simulink subsystem "TController"  (R2021a)
settings: Solver=VariableStepAuto  StartTime=0.0  StopTime=10.0  RelTol=1e-3
(part 1 of 2)
settings Model: Creator=phill  LastModifiedBy=phill

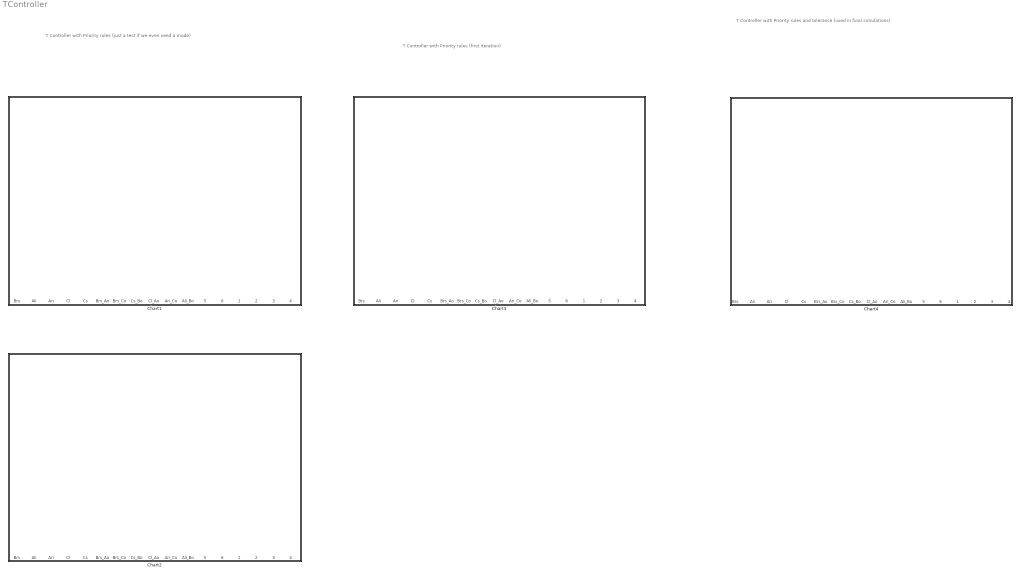
== system TController ==
  note: T Controller with Priority rules (first iteration)
  note: T Controller with Priority rules (just a test if we even need a mode)
  note: T Controller with Priority rules and tolerance
      | (used in final simulations)
  Chart1 : Stateflow chart  TreatAsAtomicUnit=on
      settings: PortSchema="{\"entries\":[{\"content\":{\"sides\":[{\"content\":{\"connectorIds\":[]},\"type\":\"ConnectorPlacement.EquallySpacedRectSide\",\"uuid\":\"dee1a780-e9dd-4205-adb9-3e9cb1ec0cd6\"},{\"content\":{\"connectorIds\":[],\"side\":\"RIGHT\"},\"type\":\"ConnectorPlacement.EquallySpacedRectSide\",\"uuid\":\"bc6af08d-2df8-4a74-93d0-032b7c1c381c\"},{\"content\":{\"connectorIds\":[],\"side\":\"TOP\"},\"type\":\"ConnectorPlacement.EquallySpacedRectSide\",\"uuid\":\"98fea325-c9fc-472d-8e1a-d846d6e99e12\"},{\"content\":{\"connectorIds\":[\"In5\",\"In1\",\"In2\",\"In3\",\"In4\",\"In11\",\"In10\",\"In9\",\"In8\",\"In7\",\"In6\",\"Out5\",\"Out6\",\"Out1\",\"Out2\",\"Out3\",\"Out4\"],\"side\":\"BOTTOM\"},\"type\":\"ConnectorPlacement.EquallySpacedRectSide\",\"uuid\":\"a092283f-ef46-48e2-a5f8-8210ac00b2f9\"}]},\"type\":\"ConnectorPlacement.EquallySpacedConnector\",\"uuid\":\"33a851aa-4180-41c0-b4bb-9b9c3be41936\"}],\"packageUris\":[\"http://schema.mathworks.com/mf0/Connector/R2020b\"],\"version\":\"1.0\"}"
  Chart2 : Stateflow chart  TreatAsAtomicUnit=on
      settings: PortSchema="{\"entries\":[{\"content\":{\"sides\":[{\"content\":{\"connectorIds\":[]},\"type\":\"ConnectorPlacement.EquallySpacedRectSide\",\"uuid\":\"dee1a780-e9dd-4205-adb9-3e9cb1ec0cd6\"},{\"content\":{\"connectorIds\":[],\"side\":\"RIGHT\"},\"type\":\"ConnectorPlacement.EquallySpacedRectSide\",\"uuid\":\"bc6af08d-2df8-4a74-93d0-032b7c1c381c\"},{\"content\":{\"connectorIds\":[],\"side\":\"TOP\"},\"type\":\"ConnectorPlacement.EquallySpacedRectSide\",\"uuid\":\"98fea325-c9fc-472d-8e1a-d846d6e99e12\"},{\"content\":{\"connectorIds\":[\"In5\",\"In1\",\"In2\",\"In3\",\"In4\",\"In11\",\"In10\",\"In9\",\"In8\",\"In7\",\"In6\",\"Out5\",\"Out6\",\"Out1\",\"Out2\",\"Out3\",\"Out4\"],\"side\":\"BOTTOM\"},\"type\":\"ConnectorPlacement.EquallySpacedRectSide\",\"uuid\":\"a092283f-ef46-48e2-a5f8-8210ac00b2f9\"}]},\"type\":\"ConnectorPlacement.EquallySpacedConnector\",\"uuid\":\"33a851aa-4180-41c0-b4bb-9b9c3be41936\"}],\"packageUris\":[\"http://schema.mathworks.com/mf0/Connector/R2020b\"],\"version\":\"1.0\"}"
  Chart3 : Stateflow chart  TreatAsAtomicUnit=on
      settings: PortSchema="{\"entries\":[{\"content\":{\"sides\":[{\"content\":{\"connectorIds\":[]},\"type\":\"ConnectorPlacement.EquallySpacedRectSide\",\"uuid\":\"dee1a780-e9dd-4205-adb9-3e9cb1ec0cd6\"},{\"content\":{\"connectorIds\":[],\"side\":\"RIGHT\"},\"type\":\"ConnectorPlacement.EquallySpacedRectSide\",\"uuid\":\"bc6af08d-2df8-4a74-93d0-032b7c1c381c\"},{\"content\":{\"connectorIds\":[],\"side\":\"TOP\"},\"type\":\"ConnectorPlacement.EquallySpacedRectSide\",\"uuid\":\"98fea325-c9fc-472d-8e1a-d846d6e99e12\"},{\"content\":{\"connectorIds\":[\"In5\",\"In1\",\"In2\",\"In3\",\"In4\",\"In11\",\"In10\",\"In9\",\"In8\",\"In7\",\"In6\",\"Out5\",\"Out6\",\"Out1\",\"Out2\",\"Out3\",\"Out4\"],\"side\":\"BOTTOM\"},\"type\":\"ConnectorPlacement.EquallySpacedRectSide\",\"uuid\":\"a092283f-ef46-48e2-a5f8-8210ac00b2f9\"}]},\"type\":\"ConnectorPlacement.EquallySpacedConnector\",\"uuid\":\"33a851aa-4180-41c0-b4bb-9b9c3be41936\"}],\"packageUris\":[\"http://schema.mathworks.com/mf0/Connector/R2020b\"],\"version\":\"1.0\"}"
  Chart4 : Stateflow chart  TreatAsAtomicUnit=on  mask{tol=0}
      mask prompts: tol "tolerance"
      settings: PortSchema="{\"entries\":[{\"content\":{\"sides\":[{\"content\":{\"connectorIds\":[]},\"type\":\"ConnectorPlacement.EquallySpacedRectSide\",\"uuid\":\"dee1a780-e9dd-4205-adb9-3e9cb1ec0cd6\"},{\"content\":{\"connectorIds\":[],\"side\":\"RIGHT\"},\"type\":\"ConnectorPlacement.EquallySpacedRectSide\",\"uuid\":\"bc6af08d-2df8-4a74-93d0-032b7c1c381c\"},{\"content\":{\"connectorIds\":[],\"side\":\"TOP\"},\"type\":\"ConnectorPlacement.EquallySpacedRectSide\",\"uuid\":\"98fea325-c9fc-472d-8e1a-d846d6e99e12\"},{\"content\":{\"connectorIds\":[\"In5\",\"In1\",\"In2\",\"In3\",\"In4\",\"In11\",\"In10\",\"In9\",\"In8\",\"In7\",\"In6\",\"Out5\",\"Out6\",\"Out1\",\"Out2\",\"Out3\",\"Out4\"],\"side\":\"BOTTOM\"},\"type\":\"ConnectorPlacement.EquallySpacedRectSide\",\"uuid\":\"a092283f-ef46-48e2-a5f8-8210ac00b2f9\"}]},\"type\":\"ConnectorPlacement.EquallySpacedConnector\",\"uuid\":\"33a851aa-4180-41c0-b4bb-9b9c3be41936\"}],\"packageUris\":[\"http://schema.mathworks.com/mf0/Connector/R2020b\"],\"version\":\"1.0\"}"

== stateflow chart TController/Chart2 ==
  note: Notizen (mal auf Deutsch):
      | wenn an einer kante etwas anliegt und keine der stärkeren kanten etwas anliegen hat,
      | und die konfliktbereiche frei sind: schalte kante frei
      | <Ali 3> wird dominiert von <Cl 7> und <Cs 8> [Kreuzungen: <Brs Co> <Cl Ao> <Cs Bo>
      | <Ari 4> wird nicht dominiert [Kreuzungen: <Brs Co>
      | <Cl 7> wird dominiert von <Brs 11> und <Brs 12> [Kreuzungen: <Brs Co> <Brs Ao><Ali Bo>
      | <Cs 8> wird nicht dominiert [Kreuzungen: <Ali Bo>
      | <Brs 11> wird dominiert von <Ali 3> und <Ari 4> [Kreuzungen: <Brs Ao> <Ali Bo> <Ari Co>*<Cl Ao>
      | <Brs 12> wird nicht dominiert [Kreuzungen: <Cl Ao>
      |
      | Anmerkung: die einflüsse Brs11 und Brs12 behindern sich nicht. da beide kanten an
      | EIN UND DEMSELBEN SEGMENT liegen, und unsere 0.5:0.5 gewichtung schon suggeriert,
      | dass sich hier die autos "spalten", können sich die autos beim "Parallelen" fließen
      | in die segmente <Brs Co> und <Brs Ao> nicht wirklich in die quere kommen. Oder selbst wenn sie es
      | tun, können wir nichts dagegen unternehmen - wenn wir einem der pfade gegenüber dem anderen
      | priorität geben, wird bei dem anderen jeweils NIE etwas fließen. Damit müssen wir wohl leben :(
      |
      | a)
      | if [Ali > 0 && Cl == 0 && Cs == 0 && Brs_Co == 0 && Cl_Ao == 0 && Cs_Bo == 0]{enableAli3=1;}
      | else {enableAli3=0;}
      | b)
      | if [Ari > 0 && Brs_Co == 0]{enableAri4=1;}
      | else {enableAri4=0;}
      | c)
      | if [Cl > 0 && Brs == 0 && Brs_Co == 0 && Brs_Ao == 0 && Ali_Bo == 0]{enableCl7=1;}
      | else {enableCl7=0;}
      | d)
      | if [Cs > 0 && Ali_Bo == 0]{enableCs8=1;}
      | else {enableCs8=0;}
      | e)
      | if [Brs > 0 && Ali == 0 && Ari == 0 && Ali_Bo == 0 && Ari_Co == 0 && Cl_Ao]{enableBrs11=1;}
      | else {enableBrs11=0;}
      | f)
      | if [Brs > 0 && Cl_Ao == 0]{enableBrs12=1;}
      | else {enableBrs12=0;}
      |
      | Anmerkung: Da es im Falle [Ali > 0 && Brs > 0 && Cl > 0] einen deadlock gibt, müssen wir uns entscheiden, wer fahren darf.
      |
      | // Brs11 soll das fahrtrecht bekommen, um den fluss entlang der geraden aufrechtzuerhalten, wenn möglich
      | if [Ari == 0 && (Ali_Bo == 0 && Ari_Co == 0 && Cl_Ao == 0)]{enableBrs11=1;}
      | else
      |
      | // falls Brs12 nicht kann, versucht Ali zu fahren. Eigentlich müsste Cl die nächstbeste Wahl sein,
      | // allerdings kann Cl im falle eines Deadlocks ohnehin nicht fließen, da wegen unserer modellierung
      | // der 1x2 kanten (bzw. 1x2 segmente) gilt "Deadlock => [Brs > 0] => [Brs12 will aktiv sein]" - und da
      | // Brs12 vorrang vor Cl7 hat, ist Cl7 in diesem szenario grundsätzlich blockiert.
      | if [Cs == 0 && (Brs_Co == 0 && Cl_Ao == 0 && Cs_Bo == 0)]{enableAli3=1;}
      | else //guess noone can make it
  note: ?
  note: Brs-11-<Brs Co>-6-Co
      | (Links will geradeaus)
  note: Brs-12-<Brs Ao>-1-Ao
      | (Links will geradeaus)
  note: Ari-4-<Ari Co>-5-Co
      | (Unten will rechts abbiegen)
  note: Cl-7-<Cl Ao>-2-Ao
      | (Rechts will links abbiegen)
  note: Cs-8-<Cl Ao>-9-Bo
      | (Rechts will geradeaus)
  note: Ali-3-<Ali Bo>-10-Bo
      | (Unten will Links abbiegen)
  note: Deadlock-Detection
  note: Anstelle der ebene für deadlock resolution konnte man den "Links will geradeaus" bereich in der reihenfolge VOR "Unten will links abbiegen" setzen. "Links will geradeaus" muss dann um eine weitere kante mit höchster priorität ergänzt werden mit einem label
      | [ (Ali > 0 && Brs > 0 && Cl > 0 ) && (Ari == 0 && Ali_Bo == 0 && Ari_Co == 0]{enableBrs11=1;}
      |
      | "Unten will links abbiegen" wird dann ebenfalls um eine Kante mit höchster priorität ergänzt mit dem Label
      | [ (Ali > 0 && Brs > 0 && Cl > 0) && (Cs_Bo == 0 && Cl_Ao == 0) && ~(enableBrs11==1)
  note: Deadlock-Resolution
  (junction 23) -> (junction 29) [order 1] : [Ari > 0 && Brs_Co == 0]{enableAri4=1;}
  (junction 29) -> (junction 36) [order 1] : [Cl > 0 && Brs == 0 && Brs_Co == 0 && Brs_Ao == 0 && Ali_Bo == 0]{enableCl7=1; }
  (junction 39) -> (junction 40) [order 1] : [Brs > 0 && Ali == 0 && Ari == 0 && Ali_Bo == 0 && Ari_Co == 0 && Cl_Ao]{enableBrs11=1;}
  (junction 40) -> (junction 45) [order 1] : [Brs > 0 && Cl_Ao == 0]{enableBrs12=1;}
  (junction 36) -> (junction 39) [order 1] : [Cs > 0 && Ali_Bo == 0]{enableCs8=1;}
  (junction 79) -> (junction 23) [order 1] : [Ali > 0 && Cl == 0 && Cs == 0 && Brs_Co == 0 && Cl_Ao == 0 && Cs_Bo == 0]
      | {enableAli3=1; }
  (junction 39) -> (junction 40) [order 2] : {enableBrs11=0;}
  (junction 79) -> (junction 23) [order 2] : {enableAli3=0;}
  (junction 29) -> (junction 36) [order 2] : {enableCl7=0;}
  (junction 36) -> (junction 39) [order 2] : {enableCs8=0;}
  (junction 23) -> (junction 29) [order 2] : {enableAri4=0;}
  (junction 40) -> (junction 45) [order 2] : {enableBrs12=0;}
  (junction 45) -> (junction 53)
  (default) -> (junction 79) : {enableAli3 = 0; enableAri4 = 0;
      | enableCl7 = 0; enableCs8 = 0;
      | enableBrs11 = 0; enableBrs12 = 0;}
  (junction 53) -> (junction 80) [order 2]
  (junction 53) -> (junction 64) [order 1] : [Ali > 0 && Brs > 0 && Cl > 0]
  (junction 71) -> (junction 80)
  (junction 64) -> (junction 71) [order 1] : [Ari == 0 && (Ali_Bo == 0 && Ari_Co == 0 && Cl_Ao == 0)]{enableBrs11=1;}
  (junction 64) -> (junction 71) [order 2] : [Ari > 0 && Cs == 0 && (Brs_Co == 0 && Cl_Ao == 0 && Cs_Bo == 0)]{enableAli3=1;}
  data: Ali input; Ari input; Cl input; Cs input; Brs input; Ali_Bo input; Ari_Co input; Cl_Ao input; Cs_Bo input; Brs_Co input; Brs_Ao input; enableAli3 output; enableAri4 output; enableCl7 output; enableCs8 output; enableBrs11 output; enableBrs12 output

== stateflow chart TController/Chart4 ==
  note: Notizen (mal auf Deutsch):
      | wenn an einer kante etwas anliegt und keine der stärkeren kanten etwas anliegen hat,
      | und die konfliktbereiche frei sind: schalte kante frei
      | <Ali 3> wird dominiert von <Cl 7> und <Cs 8> [Kreuzungen: <Brs Co> <Cl Ao> <Cs Bo>
      | <Ari 4> wird nicht dominiert [Kreuzungen: <Brs Co>
      | <Cl 7> wird dominiert von <Brs 11> und <Brs 12> [Kreuzungen: <Brs Co> <Brs Ao><Ali Bo>
      | <Cs 8> wird nicht dominiert [Kreuzungen: <Ali Bo>
      | <Brs 11> wird dominiert von <Ali 3> und <Ari 4> [Kreuzungen: <Brs Ao> <Ali Bo> <Ari Co>*<Cl Ao>
      | <Brs 12> wird nicht dominiert [Kreuzungen: <Cl Ao>
      |
      | Anmerkung: die einflüsse Brs11 und Brs12 behindern sich nicht. da beide kanten an
      | EIN UND DEMSELBEN SEGMENT liegen, und unsere 0.5:0.5 gewichtung schon suggeriert,
      | dass sich hier die autos "spalten", können sich die autos beim "Parallelen" fließen
      | in die segmente <Brs Co> und <Brs Ao> nicht wirklich in die quere kommen. Oder selbst wenn sie es
      | tun, können wir nichts dagegen unternehmen - wenn wir einem der pfade gegenüber dem anderen
      | priorität geben, wird bei dem anderen jeweils NIE etwas fließen. Damit müssen wir wohl leben :(
      |
      | a)
      | if [Ali > 0 && Cl == 0 && Cs == 0 && Brs_Co == 0 && Cl_Ao == 0 && Cs_Bo == 0]{enableAli3=1;}
      | else {enableAli3=0;}
      | b)
      | if [Ari > 0 && Brs_Co == 0]{enableAri4=1;}
      | else {enableAri4=0;}
      | c)
      | if [Cl > 0 && Brs == 0 && Brs_Co == 0 && Brs_Ao == 0 && Ali_Bo == 0]{enableCl7=1;}
      | else {enableCl7=0;}
      | d)
      | if [Cs > 0 && Ali_Bo == 0]{enableCs8=1;}
      | else {enableCs8=0;}
      | e)
      | if [Brs > 0 && Ali == 0 && Ari == 0 && Ali_Bo == 0 && Ari_Co == 0 && Cl_Ao]{enableBrs11=1;}
      | else {enableBrs11=0;}
      | f)
      | if [Brs > 0 && Cl_Ao == 0]{enableBrs12=1;}
      | else {enableBrs12=0;}
      |
      | Anmerkung: Da es im Falle [Ali > 0 && Brs > 0 && Cl > 0] einen deadlock gibt, müssen wir uns entscheiden, wer fahren darf.
      |
      | // Brs11 soll das fahrtrecht bekommen, um den fluss entlang der geraden aufrechtzuerhalten, wenn möglich
      | if [Ari == 0 && (Ali_Bo == 0 && Ari_Co == 0 && Cl_Ao == 0)]{enableBrs11=1;}
      | else
      |
      | // falls Brs12 nicht kann, versucht Ali zu fahren. Eigentlich müsste Cl die nächstbeste Wahl sein,
      | // allerdings kann Cl im falle eines Deadlocks ohnehin nicht fließen, da wegen unserer modellierung
      | // der 1x2 kanten (bzw. 1x2 segmente) gilt "Deadlock => [Brs > 0] => [Brs12 will aktiv sein]" - und da
      | // Brs12 vorrang vor Cl7 hat, ist Cl7 in diesem szenario grundsätzlich blockiert.
      | if [Cs == 0 && (Brs_Co == 0 && Cl_Ao == 0 && Cs_Bo == 0)]{enableAli3=1;}
      | else //guess noone can make it
  note: ?
  state InitiatePerStepCheck
  note: Brs-11-<Brs Co>-6-Co
      | (Links will geradeaus)
  note: Brs-12-<Brs Ao>-1-Ao
      | (Links will geradeaus)
  note: Ari-4-<Ari Co>-5-Co
      | (Unten will rechts abbiegen)
  note: Cl-7-<Cl Ao>-2-Ao
      | (Rechts will links abbiegen)
  note: Cs-8-<Cl Ao>-9-Bo
      | (Rechts will geradeaus)
  note: Ali-3-<Ali Bo>-10-Bo
      | (Unten will Links abbiegen)
  note: Deadlock-Detection
  note: Anstelle der ebene für deadlock resolution konnte man den "Links will geradeaus" bereich in der reihenfolge VOR "Unten will links abbiegen" setzen. "Links will geradeaus" muss dann um eine weitere kante mit höchster priorität ergänzt werden mit einem label
      | [ (Ali > 0 && Brs > 0 && Cl > 0 ) && (Ari == 0 && Ali_Bo == 0 && Ari_Co == 0]{enableBrs11=1;}
      |
      | "Unten will links abbiegen" wird dann ebenfalls um eine Kante mit höchster priorität ergänzt mit dem Label
      | [ (Ali > 0 && Brs > 0 && Cl > 0) && (Cs_Bo == 0 && Cl_Ao == 0) && ~(enableBrs11==1)
  note: Deadlock-Resolution
  InitiatePerStepCheck -> (junction 23) [order 1] : [Ali > 0 && Cl == 0 && Cs == 0 && Brs_Co <= tol && Cl_Ao <= tol && Cs_Bo <= tol]
      | {enableAli3=1; }
  (junction 23) -> (junction 29) [order 1] : [Ari > 0 && Brs_Co <= tol]{enableAri4=1;}
  (junction 29) -> (junction 36) [order 1] : [Cl > 0 && Brs == 0 && Brs_Co <= tol && Brs_Ao <= tol && Ali_Bo <= tol]{enableCl7=1; }
  (junction 39) -> (junction 40) [order 1] : [Brs > 0 && Ali == 0 && Ari == 0 && Ali_Bo <= tol && Ari_Co <= tol && Cl_Ao <= tol]{enableBrs11=1;}
  (junction 40) -> (junction 45) [order 1] : [Brs > 0 && Cl_Ao <= tol]{enableBrs12=1;}
  (junction 36) -> (junction 39) [order 1] : [Cs > 0 && Ali_Bo <= tol]{enableCs8=1;}
  (junction 39) -> (junction 40) [order 2] : {enableBrs11=0;}
  (junction 29) -> (junction 36) [order 2] : {enableCl7=0;}
  (junction 36) -> (junction 39) [order 2] : {enableCs8=0;}
  (junction 23) -> (junction 29) [order 2] : {enableAri4=0;}
  (junction 40) -> (junction 45) [order 2] : {enableBrs12=0;}
  InitiatePerStepCheck -> (junction 23) [order 2] : {enableAli3=0;}
  (junction 45) -> (junction 53)
  (junction 53) -> InitiatePerStepCheck [order 2]
  (default) -> InitiatePerStepCheck : {enableAli3 = 0; enableAri4 = 0;
      | enableCl7 = 0; enableCs8 = 0;
      | enableBrs11 = 0; enableBrs12 = 0;}
  (junction 53) -> (junction 64) [order 1] : [Ali > 0 && Brs > 0 && Cl > 0]
  (junction 64) -> (junction 71) [order 1] : [Ari == 0 && (Ali_Bo <= tol && Ari_Co <= tol && Cl_Ao <= tol)]{enableBrs11=1;}
  (junction 64) -> (junction 71) [order 2] : [Ari > 0 && Cs == 0 && (Brs_Co <= tol && Cl_Ao <= tol && Cs_Bo <= tol)]{enableAli3=1;}
  (junction 71) -> InitiatePerStepCheck
  data: Ali input; Ari input; Cl input; Cs input; Brs input; Ali_Bo input; Ari_Co input; Cl_Ao input; Cs_Bo input; Brs_Co input; Brs_Ao input; enableAli3 output; enableAri4 output; enableCl7 output; enableCs8 output; enableBrs11 output; enableBrs12 output; tol parameter
